simulink model "concept3_simulink_RL"  (R2025a)
settings: Solver=VariableStepAuto  StartTime=0.0  StopTime=Tf  FixedStep=0.001  MaxStep=0.01  MinStep=0.0001  RelTol=1e-3
InitFcn:
  | loaded_data = load('concept3_for_sim.mat');
  | robot = loaded_data.robot;
  | robot.DataFormat = 'column';
values from neighbouring files (symbols this model uses):
  mass = 40    [RL_main.m]    (also in baseline_sim.m)
  obs_vec = opa    [RL_main.m]    (also in baseline_sim.m)
  port = data(n, :)    [RL_main.m]    (also in baseline_sim.m = port_pos_data(n,:))
  port_num = 10    [RL_main.m]    (also in baseline_sim.m)
  port_target = AB2port(port_num)    [RL_main.m]    (also in baseline_sim.m)
  q0arm = rad2deg([-1.283; -1.622; 2.2761853; -1.8021853; 1.112; 1.859; 0.05328])    [RL_main.m]    (also in baseline_sim.m)
  q0b = [1; 0; 0; 0; 0; 0; 0]    [RL_main.m]    (also in baseline_sim.m = [1;0;0;0;0;0;0])
  sat_docked = AB2port(sat_docked_num)    [RL_main.m]    (also in baseline_sim.m)
  sat_docked_num = 6    [RL_main.m]    (also in baseline_sim.m)
  sim_state = 1    [RL_main.m]    (also in baseline_sim.m)
  Tlog = 0.1    [RL_main.m]    (also in baseline_sim.m)
  use_RL = 1    [RL_main.m]    (also in baseline_sim.m)
undefined symbols (not defined in the file or in its folder): opa, target, X, Y, Z
libraries: sm_lib x133, nesl_utility x67, simulink_extras x3, rllib x2
(part 6 of 6)

== matlab function concept3_simulink_RL/QP/MATLAB Function1 ==
  settings: updateMethod=DISCRETE  sampleTime=Tq
  data: clock input; alpha_out output
function alpha_out = alpha_star_lookup(clock)
%#codegen
% offline α*(t) 룩업 — Simulink MATLAB Function 블록
%
% 입력:
%   clock     (1×1): 시뮬레이션 절대 시간 [s]
%
% 출력:
%   alpha_out (1×1): null-space 파라미터 α*(t)
%
% 동작:
%   presim에서 계산된 전체 구간(0~Tf) α*(t)를 clock 기준으로 룩업

persistent alpha_data Ts_inv N_data t0_data

if isempty(alpha_data)
    raw        = coder.load('alpha_star_offline.mat', 'alpha_star', 'tt');
    alpha_data = raw.alpha_star;                                          % N×1
    Ts_inv     = (length(raw.tt) - 1) / (raw.tt(end) - raw.tt(1));      % 1/Ts
    N_data     = int32(length(raw.alpha_star));
    t0_data    = raw.tt(1);
end

% clock 기준 직접 인덱싱 (균일 시간축 가정)
idx = int32(round((clock - t0_data) * Ts_inv)) + int32(1);
idx = max(int32(1), min(N_data, idx));
alpha_out = alpha_data(idx);
end

== matlab function concept3_simulink_RL/Controller/MATLAB Function ==
  data: qdot_err input; Torque output
function Torque = fcn(qdot_err)
Kpgain = [500 500 500 500 50 10 10];
%Kpgain = [100 100 100 100 50  10 10];
Kp = diag(Kpgain);
Kd = diag([5,5,5,5,5,5,5]);

Torque = Kp*qdot_err;% - Kd*qdot;

== matlab function concept3_simulink_RL/QP/Path-Planning /MATLAB Function4 ==
  settings: updateMethod=DISCRETE  sampleTime=0.01
  data: ydot output; y output; clock input
function [ydot, y] = Poly_traj_homing(clock)
%#codegen
docked = 1;
% ── 웨이포인트만 여기서 수정 ──────────────────────────
%      x      y       z    roll  pitch  yaw
WP = [ 2.5   0.35    0     -90    0      -90;    % WP1 (시작)
       2.5   1.5     0     -90    0      0;    % WP2
      -0.4   1.5     0     -90    0      0;    % WP3
      -0.4   0.795   0     -90    0      0];   % WP4

T_seg = [32, 60, 20];   % 각 구간 시간 [s]
% ──────────────────────────────────────────────────────

persistent coeffs t_dock
if isempty(coeffs)
    N = length(T_seg);
    coeffs = zeros(6, 6, N);
    for s = 1:N
        T = T_seg(s);
        for d = 1:6
            dy = WP(s+1,d) - WP(s,d);
            coeffs(d,:,s) = [6*dy/T^5, -15*dy/T^4, 10*dy/T^3, 0, 0, WP(s,d)];
        end
    end
end
if isempty(t_dock); t_dock = -1.0; end

y    = zeros(6, 1, 'like', clock);
ydot = zeros(6, 1, 'like', clock);

if ~docked
    y = coeffs(:, 6, 1);
    return;
end
if t_dock < 0; t_dock = clock; end

t    = clock - t_dock;
cumT = cumsum(T_seg);
N    = length(T_seg);

% 구간 선택 — N 구간 자동 대응
seg_i = int32(N);
t0    = cumT(max(N-1, 1));
for s = 1:N
    if t < cumT(s)
        seg_i = int32(s);
        if s == 1;  t0 = 0.0;
        else;       t0 = cumT(s-1);
        end
        break;
    end
end
if t >= cumT(N);  t = cumT(N);  end   % 마지막 구간 끝 클램핑

tau = t - t0;
for d = 1:6
    a5=coeffs(d,1,seg_i); a4=coeffs(d,2,seg_i); a3=coeffs(d,3,seg_i);
    a2=coeffs(d,4,seg_i); a1=coeffs(d,5,seg_i); a0=coeffs(d,6,seg_i);
    y(d)    = ((((a5*tau+a4)*tau+a3)*tau+a2)*tau+a1)*tau+a0;
    ydot(d) = (((5*a5*tau+4*a4)*tau+3*a3)*tau+2*a2)*tau+a1;
end
ydot(4:6) = deg2rad(ydot(4:6));
end

== matlab function concept3_simulink_RL/Plant/station_robot_arm/Subsystem/MATLAB Function1 ==
  data: qe input; y output
function y = fcn(qe)

q0 = [1 0 0 0];

% 쿼터니언 dot product (절대값으로 동일 회전 처리)
dq = abs(dot(q0, qe));

% domain clipping
dq = max(min(dq, 1), -1);

% quaternion distance [deg]
thetaq = rad2deg(2 * acos(dq));

y = thetaq;

== matlab function concept3_simulink_RL/QP/Path-Planning /MATLAB Function ==
  data: pos_rpy input; EE_pos output; docked input
function EE_pos = fcn(pos_rpy, docked)
%#codegen

% -------- 1) 입력 분해 --------
pos_rpy(1:3) = pos_rpy(1:3) - [1.35; 0.225; 0.325];
p = pos_rpy(1:3).';
rpy_deg = pos_rpy(4:6).';
eulZYX_rad = deg2rad([rpy_deg(3), rpy_deg(2), rpy_deg(1)]);

% -------- 2) 베이스->타깃포트 변환행렬 --------
T_base_to_target = eul2tform(eulZYX_rad, 'ZYX');
T_base_to_target(1:3,4) = p(:);

% -------- 3) EE 타깃 포즈 계산 --------
if docked
    % 도킹 완료: 그리퍼 끝단 오프셋 없이 EE 포즈 = 포트 포즈
    T_base_to_ee = T_base_to_target;
else
    % 미도킹: 툴 오프셋 역적용
    T_roll       = eul2tform([0, 0, pi], 'ZYX');
    T_trans      = trvec2tform([0, 0, -0.505]);
    T_ee_to_tool = T_roll * T_trans;
    T_base_to_ee = T_base_to_target / T_ee_to_tool;
end

% -------- 4) 변환행렬 -> [pos; RPY(deg)] --------
pos         = tform2trvec(T_base_to_ee).';
eulZYX_out  = tform2eul(T_base_to_ee, 'ZYX');
rpy_out_deg = rad2deg([eulZYX_out(3); eulZYX_out(2); eulZYX_out(1)]);

EE_pos = [pos; rpy_out_deg];
end

== matlab function concept3_simulink_RL/Plant/Attach_logic/Attach sensor/Subsystem/Quat2RPY ==
  data: q_current input; RPY output
function RPY = fcn(q_current)

sequence = 'ZYX';

eul_angles_rad_out = quat2eul(q_current', sequence);

%eul_angles_deg_out = rad2deg(eul_angles_rad_out);

yaw_out = eul_angles_rad_out(1);
pitch_out = eul_angles_rad_out(2);
roll_out = eul_angles_rad_out(3);

RPY = [roll_out; pitch_out; yaw_out];

== matlab function concept3_simulink_RL/R2L/reward1 ==
  data: EE_err input; ori_err input; tau input; done input; r output; r_el output; donebad input
function [r, r_el] = reward_fn(EE_err, ori_err, tau, done, donebad)
    % 1. 외부 함수 호출 선언
    coder.extrinsic('reward_fn');
    
    % 2. 출력 변수 크기 및 타입 사전 할당 (Pre-allocation)
    % Simulink 컴파일러가 출력 형태를 미리 알 수 있도록 함
    r = 0.0;                 % 스칼라
    r_el = zeros(1, 4);      % 1x4 벡터
    
    % 3. 외부 스크립트 실행
    [r, r_el] = reward_fn(EE_err, ori_err, tau, done, donebad);
end

== matlab function concept3_simulink_RL/QP/CLIK1/Quat2RPY ==
  data: q_current input; RPY output
function RPY = fcn(q_current)

sequence = 'ZYX';

eul_angles_rad_out = quat2eul(q_current', sequence);

eul_angles_deg_out = rad2deg(eul_angles_rad_out);

yaw_deg_out = eul_angles_deg_out(1);
pitch_deg_out = eul_angles_deg_out(2);
roll_deg_out = eul_angles_deg_out(3);

RPY = [roll_deg_out; pitch_deg_out; yaw_deg_out];

== matlab function concept3_simulink_RL/QP1/CLIK/quaternion sum ==
  data: q_target_RPY input; e_rot output; q_current input
function e_rot = fcn(q_target_RPY,q_current)

roll_rad = deg2rad(q_target_RPY(1));
pitch_rad = deg2rad(q_target_RPY(2));
yaw_rad = deg2rad(q_target_RPY(3));

sequence = 'ZYX';

eul_angles_rad = [yaw_rad, pitch_rad, roll_rad];
q_target = eul2quat(eul_angles_rad, sequence);

if dot(q_target, q_current) < 0
    q_current = -q_current;
end

% 오차 쿼터니언 계산
q_current_conj = [q_current(1), -q_current(2), -q_current(3), -q_current(4)];

% 쿼터니언 곱(quatmultiply) 직접 구현
w1 = q_target(1); 
x1 = q_target(2); 
y1 = q_target(3); 
z1 = q_target(4);

w2 = q_current_conj(1); 
x2 = q_current_conj(2); 
y2 = q_current_conj(3); 
z2 = q_current_conj(4);

w_err = w1*w2 - x1*x2 - y1*y2 - z1*z2;
x_err = w1*x2 + x1*w2 + y1*z2 - z1*y2;
y_err = w1*y2 - x1*z2 + y1*w2 + z1*x2;
z_err = w1*z2 + x1*y2 - y1*x2 + z1*w2;

q_err = [w_err, x_err, y_err, z_err];


% 3차원 오차 벡터 추출
e_rot = q_err(2:4)'; % 3x1 컬럼 벡터로 변환

== matlab function concept3_simulink_RL/QP1/MATLAB Function ==
  data: pos_rpy input; EE_pos output
function EE_pos = fcn(pos_rpy)
%#codegen
% Input : pos_rpy = [x; y; z; roll; pitch; yaw]  (deg, ZYX: roll(X)-pitch(Y)-yaw(Z))
% Output: EE_pos  = [x; y; z; roll; pitch; yaw] (deg, ZYX)
%
% 역할:
%  - 주어진 "타깃 포트"의 포즈(베이스 기준)를 입력으로 받아
%  - 툴 오프셋(roll 180deg + 그 프레임의 Z-방향으로 -0.315m)을 역적용해서
%  - 로봇 EE가 가져야 할 포즈(베이스 기준)를 반환

% -------- 1) 입력 분해 --------
pos_rpy(1:3) = pos_rpy(1:3)-[1.35; 0.225; 0.325]; % 로봇팔 베이스 빼기 
p = pos_rpy(1:3).';             % [x y z]
rpy_deg = pos_rpy(4:6).';       % [roll pitch yaw] (deg, ZYX)

% eul2tform('ZYX')는 입력이 [yaw pitch roll] 순(라디안)
eulZYX_rad = deg2rad([rpy_deg(3), rpy_deg(2), rpy_deg(1)]);

% -------- 2) 베이스->타깃포트 변환행렬 만들기 --------
T_base_to_target = eul2tform(eulZYX_rad, 'ZYX');  % 회전
T_base_to_target(1:3,4) = p(:);                   % 위치

% -------- 3) 툴 오프셋(EE->툴) 정의 --------
%  - 툴 프레임은 EE 프레임에서 X축(roll)으로 180deg 회전한 뒤,
%    그 회전된 Z축 방향으로 -0.315m 떨어져 있다고 가정
T_roll = eul2tform([0, 0, pi], 'ZYX');        % roll 180 deg
T_trans = trvec2tform([0, 0, -0.510]);       % 그 프레임의 +Z로 -0.315m
T_ee_to_tool = T_roll * T_trans;             % 회전 후 이동

% -------- 4) EE 타깃 포즈 계산 --------
%  타깃 포트 포즈 = EE 포즈 * (EE->툴)
%  => EE 포즈 = 타깃 포즈 * (EE->툴)^-1
T_base_to_ee = T_base_to_target / T_ee_to_tool;

% -------- 5) 변환행렬 -> [pos; RPY(deg)]로 변환 --------
pos = tform2trvec(T_base_to_ee).';
eulZYX_out = tform2eul(T_base_to_ee, 'ZYX');   % [yaw pitch roll] (rad)
rpy_out_deg = rad2deg([eulZYX_out(3); eulZYX_out(2); eulZYX_out(1)]);

EE_pos = [pos; rpy_out_deg];
end

== matlab function concept3_simulink_RL/QP/CLIK1/quaternion sum ==
  data: q_target_RPY input; e_rot output; q_current input
function e_rot = fcn(q_target_RPY,q_current)

roll_rad = deg2rad(q_target_RPY(1));
pitch_rad = deg2rad(q_target_RPY(2));
yaw_rad = deg2rad(q_target_RPY(3));

sequence = 'ZYX';

eul_angles_rad = [yaw_rad, pitch_rad, roll_rad];
q_target = eul2quat(eul_angles_rad, sequence);

if dot(q_target, q_current) < 0
    q_current = -q_current;
end

% 오차 쿼터니언 계산
q_current_conj = [q_current(1), -q_current(2), -q_current(3), -q_current(4)];

% 쿼터니언 곱(quatmultiply) 직접 구현
w1 = q_target(1); 
x1 = q_target(2); 
y1 = q_target(3); 
z1 = q_target(4);

w2 = q_current_conj(1); 
x2 = q_current_conj(2); 
y2 = q_current_conj(3); 
z2 = q_current_conj(4);

w_err = w1*w2 - x1*x2 - y1*y2 - z1*z2;
x_err = w1*x2 + x1*w2 + y1*z2 - z1*y2;
y_err = w1*y2 - x1*z2 + y1*w2 + z1*x2;
z_err = w1*z2 + x1*y2 - y1*x2 + z1*w2;

q_err = [w_err, x_err, y_err, z_err];


% 3차원 오차 벡터 추출
e_rot = q_err(2:4)'; % 3x1 컬럼 벡터로 변환

== matlab function concept3_simulink_RL/R2L/reward ==
  data: EE_err input; ori_err input; tau input; done input; r output; r_el output; donebad input
function [r,r_el] = reward_fn(EE_err, ori_err, tau, done, donebad)
% --------------------------------------------
% Multi-objective Gaussian Reward Function
% EE_err : end-effector position error [m]
% ori_err : base attitude quaternion error [deg]
% tau : 7x1 joint torque vector
% done : terminal flag
% --------------------------------------------

%% ====== Hyperparameters (σ 값들) ======
sigma_EE   = 0.04;    % EE 오차 1cm 정도가 acceptable
sigma_ori  = 14;       % 5 deg 이하면 양호
sigma_tau  = 3;       % 토크 5 Nm 정도 허용 (로봇팔 스펙 따라 조정)
sigma_final = 2;      % 최종자세는 더 엄격하게 (2 deg)

%% ====== 개별 Gaussian 보상 ======

% 1) EE 추종 보상
R_ee = exp( - (EE_err^2) / (2*sigma_EE^2) );

% 2) Base Orientation 보상 (degree)
R_ori = exp( - (ori_err^2) / (2*sigma_ori^2) );

% 3) Torque penalty (7×1)
tau_norm = norm(tau);
R_tau = exp( - (tau_norm^2) / (2*sigma_tau^2) );

%% ====== Terminal Reward ======
if done == 1
    % 최종 자세는 훨씬 강한 패널티
    P_final = -(10-ori_err)^2;
else
    P_final = 0;
end

if donebad
    P_bad = -40;
else
    P_bad = 0;
end


%% ====== Gaussian squash (논문 스타일) ======
sigma1 = 0.5;   % EE term sensitivity   작을수록 민감
sigma2 = 0.5;   % Orientation term sensitivity
sigma3 = 0.5;   % Torque term sensitivity

G_ee  = -exp(-abs(R_ee)  / sigma1);
G_ori = -exp(-abs(R_ori) / sigma2);
G_tau = -exp(-abs(R_tau) / sigma3);

%% ====== 가중 합성 / 최종 보상 ======
w1 = 1.0;  % EE
w2 = 2.0;  % Orientation
w3 = 1.0;  % Torque
w4 = 1.0;  % Terminal term

r = w1*G_ee + w2*G_ori + w3*G_tau + w4*P_final+P_bad;

%% ====== 요소별 출력 ======
r_el = [w1*G_ee  w2*G_ori w3*G_tau w4*P_final];
end
